simulink model "Induction_motor_Starter_testing"  (R2024a)
settings: Solver=VariableStepAuto  StartTime=0.0  StopTime=10  RelTol=1e-3
libraries: spsACVoltageSourceLib x3, spsThreePhaseBreakerLib x3, spsThreePhaseVIMeasurementLib x2, spsAsynchronousMachineSIUnitsLib x1, spsGroundLib x1, simulink x1, simulink_extras x1, sps_lib x1
settings Model: Creator=gshma  LastModifiedBy=gshma

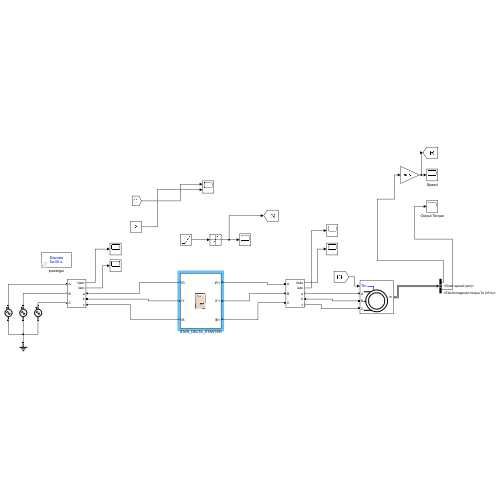
[thumbnail: Simulink's stored preview of the top-level diagram]
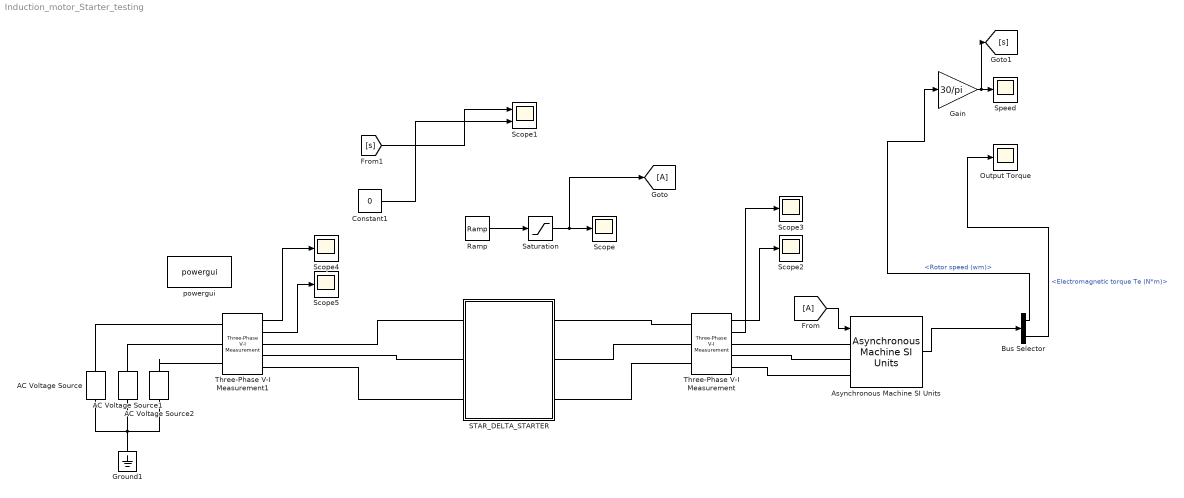
== system Induction_motor_Starter_testing ==
  AC Voltage Source : spsACVoltageSourceLib/AC Voltage Source  Amplitude=400/sqrt(3)  Phase=0  Frequency=50  SampleTime=0  Measurements=None  BusType=swing  Pref=10e3  Qref=0  Qmin=-inf  Qmax=+inf
  AC Voltage Source1 : spsACVoltageSourceLib/AC Voltage Source  Amplitude=400/sqrt(3)  Phase=120  Frequency=50  SampleTime=0  Measurements=None  BusType=swing  Pref=10e3  Qref=0  Qmin=-inf  Qmax=+inf
  AC Voltage Source2 : spsACVoltageSourceLib/AC Voltage Source  Amplitude=400/sqrt(3)  Phase=240  Frequency=50  SampleTime=0  Measurements=None  BusType=swing  Pref=10e3  Qref=0  Qmin=-inf  Qmax=+inf
  Asynchronous Machine SI Units : spsAsynchronousMachineSIUnitsLib/Asynchronous Machine SI Units  RotorType=Squirrel-cage  PresetModel="15:  5.4 HP (4KW)   400 V  50Hz 1430 RPM"  MechanicalLoad=Torque Tm  ShowDetailedParameters=on  ReferenceFrame=Rotor  Units=SI  MeasurementBus=off  NominalParameters=[4000 400 50]  VoltageRatio=1  Stator=[1.405 0.005839]  Rotor=[1.395 0.005839]  Cage1=[0.4155 0.002066]  Cage2=[0.4168 0.0003495]  Lm=0.1722  Mechanical=[0.0131 0.002985 2]  PolePairs=2  InitialConditions=[0.05 0 0 0 0 0 0 0]  SimulateSaturation=off  Saturation=[14.03593122, 27.81365428, 53.79336849, 72.68890987, 97.98006896, 148.6815601, 215.7428561, 302.9841135, 428.7778367 ; 230, 322, 414, 460, 506, 552, 598, 644, 690]  LoadFlowParameters=1492000  TsPowergui=0  TsBlock=-1  IterativeModel=Trapezoidal non iterative  IterativeDiscreteModel=Trapezoidal non iterative  Pmec=1.492e+006
  Bus Selector : BusSelector  OutputSignals=Mechanical.Rotor speed (wm),Mechanical.Electromagnetic torque Te (N*m)
  Constant1 : Constant  Value=0  OutDataTypeStr=boolean  SampleTime=0.001
  From : From
  Gain : Gain  Gain=30/pi
  Goto : Goto
  Ground1 : spsGroundLib/Ground  LConnTagsString=a
  Output Torque : Scope
  Ramp : simulink/Sources/Ramp  slope=5  start=0.9  InitialOutput=0
  STAR_DELTA_STARTER : Subsystem
      mask Display: image('star_delt.jpg', [0,0,0,0,50,50]);
  Saturation : Saturate  UpperLimit=26.5  LowerLimit=1
  Scope{,2..5} (5 alike) : Scope
  Scope1 : Scope  NumInputPorts=2
  Speed : Scope
  Three-Phase V-I Measurement : spsThreePhaseVIMeasurementLib/Three-Phase V-I Measurement  VoltageMeasurement=phase-to-phase  SetLabelV=off  LabelV=Vabc  Vpu=off  VpuLL=off  CurrentMeasurement=yes  SetLabelI=off  LabelI=Iabc  Ipu=off  Pbase=100e6  Vbase=500e3  OutputType=Complex  PhasorSimulation=off  PSBequivalent=0
  Three-Phase V-I Measurement1 : spsThreePhaseVIMeasurementLib/Three-Phase V-I Measurement  VoltageMeasurement=phase-to-phase  SetLabelV=off  LabelV=Vabc  Vpu=off  VpuLL=off  CurrentMeasurement=yes  SetLabelI=off  LabelI=Iabc  Ipu=off  Pbase=100e6  Vbase=500e3  OutputType=Complex  PhasorSimulation=off  PSBequivalent=0
  powergui : sps_lib/powergui  Priority=1  SimulationMode=Discrete  SampleTime=50e-6  frequency=60  Iterations=50  frequencyindice=50  Pbase=100e6  ErrMax=1e-4  UnitsV=kV  UnitsW=MW  buscounter=0  FunctionMessages=off  echomessages=off  EnableUseOfTLC=off  CurrentSourceSwitches=off  DisableSnubberDevices=off  DisableRonSwitches=off  DisableVfSwitches=off  DisplayEquations=off  AutomaticDiscreteSolvers=off  SolverType=Tustin/Backward Euler (TBE)  Interpol=off  ExternalGateDelay=off  methode=off  Ts=100  x0status=blocks  SPID=on  SwTol=0  HookPort=off  NonlinearTolerance=1e-4  nMaxIteration=100  ContinueOnMaxIteration=off  RestoreLinks=warning  ResistiveCurrentMeasurement=off  Frange=[0:2:500]  Ylog=off  Xlog=on  ShowGrid=off  save=off  variable=ZData  structure=0  ZoomFFT=off  StartTime=0.0  cycles=1  DisplayStyle=1  fundamental=60  FreqAxis=off  MaxFrequency=1000  frequencyindicesteady=1  RmsSteady=1  display=off
  wires:
  Asynchronous Machine SI Units/1 -> Bus Selector/1
  Bus Selector/1 -> Gain/1  "<Rotor speed (wm)>"
  Gain/1 -> [s], Speed/1
  Bus Selector/2 -> Output Torque/1  "<Electromagnetic torque Te (N*m)>"
  From/1 -> Asynchronous Machine SI Units/1
  Three-Phase V-I Measurement/2 -> Scope3/1
  Three-Phase V-I Measurement/1 -> Scope2/1
  Three-Phase V-I Measurement1/1 -> Scope4/1
  Three-Phase V-I Measurement1/2 -> Scope5/1
  Ramp/1 -> Saturation/1
  Saturation/1 -> Goto/1, Scope/1
  [s] -> Scope1/1
  Constant1/1 -> Scope1/2
  connections:
  Three-Phase V-I Measurement/RConn1 -- Asynchronous Machine SI Units/LConn1
  Three-Phase V-I Measurement/RConn2 -- Asynchronous Machine SI Units/LConn2
  Three-Phase V-I Measurement/RConn3 -- Asynchronous Machine SI Units/LConn3
  Three-Phase V-I Measurement1/RConn2 -- STAR_DELTA_STARTER/LConn2
  Three-Phase V-I Measurement1/RConn3 -- STAR_DELTA_STARTER/LConn3
  Three-Phase V-I Measurement1/RConn1 -- STAR_DELTA_STARTER/LConn1
  STAR_DELTA_STARTER/RConn1 -- Three-Phase V-I Measurement/LConn1
  Three-Phase V-I Measurement/LConn2 -- STAR_DELTA_STARTER/RConn2
  Three-Phase V-I Measurement/LConn3 -- STAR_DELTA_STARTER/RConn3
  AC Voltage Source1/LConn1 -- AC Voltage Source/LConn1 -- AC Voltage Source2/LConn1 -- Ground1/LConn1
  AC Voltage Source1/RConn1 -- Three-Phase V-I Measurement1/LConn2
  AC Voltage Source2/RConn1 -- Three-Phase V-I Measurement1/LConn3
  AC Voltage Source/RConn1 -- Three-Phase V-I Measurement1/LConn1

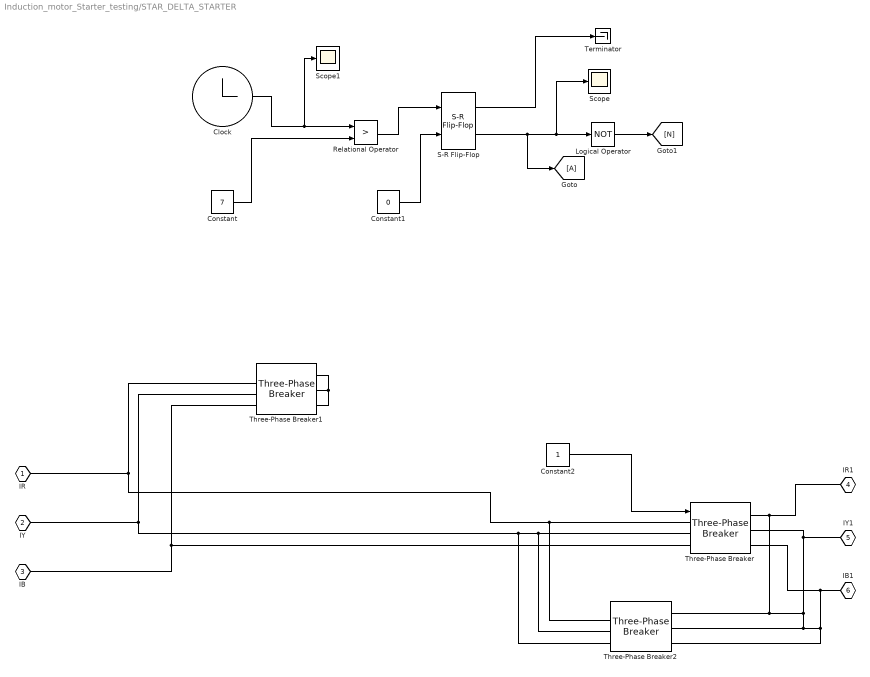
== system Induction_motor_Starter_testing/STAR_DELTA_STARTER ==
  Clock : Clock
      settings: Decimation=1000
  Constant : Constant  Value=7  SampleTime=0.001
  Constant1 : Constant  Value=0  OutDataTypeStr=boolean  SampleTime=0.0001
  Constant2 : Constant  OutDataTypeStr=boolean
  Goto : Goto
  Logical Operator : Logic  Operator=NOT  AllPortsSameDT=off  OutDataTypeStr=boolean
  Relational Operator : RelationalOperator  Operator=>  OutDataTypeStr=boolean  RndMeth=Simplest  InputSameDT=off
  S-R Flip-Flop : simulink_extras/Flip Flops/S-R Flip-Flop  initial_condition=0
  Scope : Scope
  Scope1 : Scope
  Terminator : Terminator
  Three-Phase Breaker : spsThreePhaseBreakerLib/Three-Phase Breaker  InitialState=closed  SwitchA=on  SwitchB=on  SwitchC=on  SwitchTimes="[1/60  5/60]"  External=on  BreakerResistance=0.01  SnubberResistance=1e6  SnubberCapacitance=inf  Measurements=None
  Three-Phase Breaker1 : spsThreePhaseBreakerLib/Three-Phase Breaker  InitialState=closed  SwitchA=on  SwitchB=on  SwitchC=on  SwitchTimes="[1/60  5/60]"  External=on  BreakerResistance=0.01  SnubberResistance=1e6  SnubberCapacitance=inf  Measurements=None
  Three-Phase Breaker2 : spsThreePhaseBreakerLib/Three-Phase Breaker  InitialState=closed  SwitchA=on  SwitchB=on  SwitchC=on  SwitchTimes="[1/60  5/60]"  External=on  BreakerResistance=0.01  SnubberResistance=1e6  SnubberCapacitance=inf  Measurements=None
  IR : PMIOPort  Tag=simrfV2util1/Connection Port  Side=Left
  IY : PMIOPort  Tag=simrfV2util1/Connection Port  Port=2  Side=Left
  IB : PMIOPort  Tag=simrfV2util1/Connection Port  Port=3  Side=Left
  IR1 : PMIOPort  Tag=simrfV2util1/Connection Port  Port=4  Side=Right
  IY1 : PMIOPort  Tag=simrfV2util1/Connection Port  Port=5  Side=Right
  IB1 : PMIOPort  Tag=simrfV2util1/Connection Port  Port=6  Side=Right
  wires:
  Relational Operator/1 -> S-R Flip-Flop/1
  S-R Flip-Flop/1 -> Terminator/1
  Constant/1 -> Relational Operator/2
  Constant1/1 -> S-R Flip-Flop/2
  Clock/1 -> Scope1/1, Relational Operator/1
  S-R Flip-Flop/2 -> Goto/1, Scope/1, Logical Operator/1
  Logical Operator/1 -> [N]
  Constant2/1 -> Three-Phase Breaker/1
  connections:
  Three-Phase Breaker/LConn1 -- Three-Phase Breaker2/LConn1 -- Three-Phase Breaker1/LConn1 -- IR/RConn1
  Three-Phase Breaker/LConn2 -- Three-Phase Breaker2/LConn2 -- Three-Phase Breaker2/LConn3 -- IY/RConn1 -- Three-Phase Breaker1/LConn2
  Three-Phase Breaker/LConn3 -- IB/RConn1 -- Three-Phase Breaker1/LConn3
  Three-Phase Breaker/RConn1 -- Three-Phase Breaker2/RConn1 -- Three-Phase Breaker2/RConn2 -- Three-Phase Breaker2/RConn3 -- Three-Phase Breaker/RConn3 -- IB1/RConn1 -- Three-Phase Breaker/RConn2 -- IY1/RConn1 -- IR1/RConn1
  Three-Phase Breaker1/RConn1 -- Three-Phase Breaker1/RConn3 -- Three-Phase Breaker1/RConn2
